simulink model "SchemaBloc"  (R2015b)
settings: Solver=FixedStepAuto  StartTime=0.0  StopTime=0.5  FixedStep=0.0001  RelTol=1e-3
values from neighbouring files (symbols this model uses):
  f = 0.2*10^(-2)    (= 0.002)    [constantes.m]
  Jeq2 = 7*10^(-3)    (= 0.007)    [constantes.m]
  Kc = 1.3    [constantes.m]
  Ke = 1.3    [constantes.m]
  L = 0.009    [constantes.m]
  R = 3    [constantes.m]
settings Model: Creator=pt_ptsi  LastModifiedBy=pt_ptsi

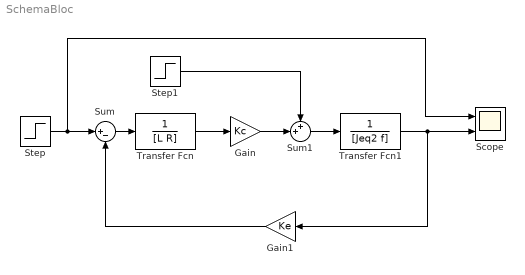
== system SchemaBloc ==
  Gain : Gain  Gain=Kc
  Gain1 : Gain  Gain=Ke
  Scope : Scope  NumInputPorts=2
  Step : Step  Time=0  SampleTime=0
  Step1 : Step  After=0  SampleTime=0
  Sum : Sum  Inputs=|+-
  Sum1 : Sum  Inputs=++|
  Transfer Fcn : TransferFcn  Denominator=[L R]
  Transfer Fcn1 : TransferFcn  Denominator=[Jeq2 f]
  wires:
  Sum/1 -> Transfer Fcn/1
  Sum1/1 -> Transfer Fcn1/1
  Step1/1 -> Sum1/1
  Gain/1 -> Sum1/2
  Transfer Fcn/1 -> Gain/1
  Transfer Fcn1/1 -> Gain1/1, Scope/2
  Step/1 -> Scope/1, Sum/1
  Gain1/1 -> Sum/2
